simulink model "ramadan_2022"  (R2021a)
settings: Solver=ode15s  StartTime=0.0  StopTime=10  MaxStep=1e-2  MinStep=1e-20  RelTol=1e-3
StartFcn:
  | tic
StopFcn:
  | toc
  | 
  | 
  | %if GimbalLockFlag
  |  % fprintf(2, 'Almost reached Gimbal Lock of IMU. Simulation stopped.\n')
  | %end
  | 
  | %fprintf('Elapsed time: %4.2f sec (%4.2f%% realtime)\n', a, tout(end)/a*100)
values from neighbouring files (symbols this model uses):
  Balance = pMod(26:29)    [AssignSimulinkParams.m]    (also in assign_parameters.m = param(26:29))
  BalanceTrunkLat = pMod(22:25)    [AssignSimulinkParams.m]    (also in assign_parameters.m = param(22:25))
  BasisStim = pMod(1:11)    [AssignSimulinkParams.m]    (also in assign_parameters.m = param(1:11))
  CompliantLeg = pMod(12:14)    [AssignSimulinkParams.m]    (also in assign_parameters.m = param(12:14))
  CompliantLegLat = pMod(15)    [AssignSimulinkParams.m]    (also in assign_parameters.m = param(15))
  lp1 = 0.45    [nms3D_prep.m]
  lp2 = 0.55    [nms3D_prep.m]
  N = size(x,1)    [cmaes_hg.m]
  PreventKneeOverextension = pMod(16:21)    [AssignSimulinkParams.m]    (also in assign_parameters.m = param(16:21))
  propulsion = pMod(35)    [AssignSimulinkParams.m]    (also in assign_parameters.m = param(35))
  s = x(1:N-1,:).^2 + x(2:N,:).^2    [cmaes_hg.m]
  Target02 = pMod(30)    [AssignSimulinkParams.m]    (also in assign_parameters.m = param(30))
  Target13 = pMod(31:33)    [AssignSimulinkParams.m]    (also in assign_parameters.m = param(31:33))
  theta0 = pMod(34)    [AssignSimulinkParams.m]    (also in assign_parameters.m = param(34))
  WramameiSL_1000 = readmatrix('WSL_1000_Norm_Sigmoid_MSE_cont.csv')    [nms3D_prep.m]
  ZramameiSL_1000 = readmatrix('ZSL_1000_Norm_Sigmoid_MSE_cont.csv')    [nms3D_prep.m]
undefined symbols (not defined in the file or in its folder): ICs, mParams, X, Y, Z
libraries: nesl_utility x110, sm_lib x88, simulink x79, eeGeneralControl x28, robotmaniplib x10, dspinverses x10, robotcorelib x5, dspmathops x3, pid_lib x2, vrlib x1
(part 9 of 9)

== system ramadan_2022/Supraspinal Level/Subsystem/Swing Leg/Compute Acceleration Profiles with Minimal Jerk Approach1/Minimal jerk Leg Angle/Minimal Jerk ==
  t : Inport
  a [6x1] : Inport  Port=2
  Add : Sum  Inputs=3
  Constant1 : Constant
  Constant3 : Constant  Value=2
  Demux : Demux  Outputs=6
  Divide3 : Product  Inputs=**
  Divide4 : Product  Inputs=**
  Divide5 : Product  Inputs=**
  Gain : Gain  Gain=60
  Gain1 : Gain  Gain=24
  Gain2 : Gain  Gain=6
  Math Function4 : Math  Operator=pow  SaturateOnIntegerOverflow=on
  Terminator : Terminator
  Terminator1 : Terminator
  Terminator2 : Terminator
  j(t) : Outport
  wires:
  a [6x1]/1 -> Demux/1
  Constant3/1 -> Math Function4/2
  Add/1 -> j(t)/1
  Demux/4 -> Divide3/2
  t/1 -> Divide4/1, Math Function4/1
  Demux/5 -> Divide4/2
  Demux/6 -> Divide5/2
  Demux/1 -> Terminator/1
  Demux/2 -> Terminator1/1
  Divide3/1 -> Gain2/1
  Divide4/1 -> Gain1/1
  Divide5/1 -> Gain/1
  Gain/1 -> Add/3
  Gain1/1 -> Add/2
  Gain2/1 -> Add/1
  Math Function4/1 -> Divide5/1
  Constant1/1 -> Divide3/1
  Demux/3 -> Terminator2/1

== system ramadan_2022/Supraspinal Level/Subsystem/Swing Leg/Compute Acceleration Profiles with Minimal Jerk Approach1/Minimal jerk Leg Angle/Minimal Jerk Parameters [Movellan] ==
  x0 : Inport
  dx0 : Inport  Port=2
  ddx0 : Inport  Port=3
  xT : Inport  Port=4
  dxT : Inport  Port=5
  ddxT : Inport  Port=6
  T : Inport  Port=7
  Demux : Demux  Outputs=3
  Gain : Gain  Gain=0.5
  Gain1 : Gain  Gain=3
  Gain2 : Gain  Gain=6
  Gain3 : Gain  Gain=4
  Gain4 : Gain  Gain=12
  Gain5 : Gain  Gain=5
  Gain6 : Gain  Gain=20
  Matrix Multiply : Product  Multiplication=Matrix(*)
  Minus : Sum  Inputs=+---
  Minus1 : Sum  Inputs=+--
  Minus2 : Sum  Inputs=+-
  Mux : Mux  Inputs=6
  Mux{1..4} (4 alike) : Mux  Inputs=3
  Pseudoinverse : dspinverses/Pseudoinverse  wanterr=off  SimulateUsing=Code generation
      settings: SourceProductBaseCode=DS
  T{2..5} (4 alike) : Product  Inputs=**
  b : Concatenate  NumInputs=3  Mode=Multidimensional array  ConcatenateDimension=2
  multiply : Product  Inputs=**
  multiply1 : Product  Inputs=**
  multiply2 : Product  Inputs=**
  a : Outport
  wires:
  xT/1 -> Minus/1
  Minus1/1 -> Mux4/2
  T5/1 -> Mux3/1
  multiply1/1 -> Minus1/3
  Gain5/1 -> Mux3/2
  Demux/2 -> Mux/5
  dxT/1 -> Minus1/1
  Demux/3 -> Mux/6
  b/1 -> Pseudoinverse/1
  multiply2/1 -> Minus/3
  Minus2/1 -> Mux4/3
  Gain/1 -> multiply/1, Mux/3
  multiply/1 -> Minus/4
  ddxT/1 -> Minus2/1
  Gain4/1 -> Mux2/3
  Gain6/1 -> Mux3/3
  x0/1 -> Minus/2, Mux/1
  Mux1/1 -> b/1
  Matrix Multiply/1 -> Demux/1
  ddx0/1 -> Minus2/2, multiply1/1, Gain/1
  T2/1 -> Gain1/1, Gain4/1, T3/1, multiply/2
  Gain2/1 -> Mux1/3
  Mux4/1 -> Matrix Multiply/2
  T4/1 -> Mux2/1, Gain5/1, T5/1
  Minus/1 -> Mux4/1
  Pseudoinverse/1 -> Matrix Multiply/1
  Mux2/1 -> b/2
  Gain3/1 -> Mux2/2
  Mux3/1 -> b/3
  Gain1/1 -> Mux1/2
  T/1 -> multiply2/2, multiply1/2, Gain2/1, T5/2, T4/2, T3/2, T2/2, T2/1
  Demux/1 -> Mux/4
  Mux/1 -> a/1
  T3/1 -> Gain6/1, Gain3/1, Mux1/1, T4/1
  dx0/1 -> multiply2/1, Minus1/2, Mux/2

== system ramadan_2022/Supraspinal Level/Subsystem/Swing Leg/Compute Acceleration Profiles with Minimal Jerk Approach1/Minimal jerk Leg Length/Enabled Subsystem ==
  In1 : Inport
  Enable : EnablePort
  Out1 : Outport  VectorParamsAs1DForOutWhenUnconnected=off
  wires:
  In1/1 -> Out1/1

== system ramadan_2022/Supraspinal Level/Subsystem/Swing Leg/Compute Acceleration Profiles with Minimal Jerk Approach1/Minimal jerk Leg Length/Minimal Jerk ==
  t : Inport
  a [6x1] : Inport  Port=2
  Add : Sum  Inputs=3
  Constant1 : Constant
  Constant3 : Constant  Value=2
  Demux : Demux  Outputs=6
  Divide3 : Product  Inputs=**
  Divide4 : Product  Inputs=**
  Divide5 : Product  Inputs=**
  Gain : Gain  Gain=60
  Gain1 : Gain  Gain=24
  Gain2 : Gain  Gain=6
  Math Function4 : Math  Operator=pow  SaturateOnIntegerOverflow=on
  Terminator : Terminator
  Terminator1 : Terminator
  Terminator2 : Terminator
  j(t) : Outport
  wires:
  a [6x1]/1 -> Demux/1
  Constant3/1 -> Math Function4/2
  Add/1 -> j(t)/1
  Demux/4 -> Divide3/2
  t/1 -> Divide4/1, Math Function4/1
  Demux/5 -> Divide4/2
  Demux/6 -> Divide5/2
  Demux/1 -> Terminator/1
  Demux/2 -> Terminator1/1
  Divide3/1 -> Gain2/1
  Divide4/1 -> Gain1/1
  Divide5/1 -> Gain/1
  Gain/1 -> Add/3
  Gain1/1 -> Add/2
  Gain2/1 -> Add/1
  Math Function4/1 -> Divide5/1
  Constant1/1 -> Divide3/1
  Demux/3 -> Terminator2/1

== system ramadan_2022/Supraspinal Level/Subsystem/Swing Leg/Compute Acceleration Profiles with Minimal Jerk Approach1/Minimal jerk Leg Length/Minimal Jerk Parameters [Movellan] ==
  x0 : Inport
  dx0 : Inport  Port=2
  ddx0 : Inport  Port=3
  xT : Inport  Port=4
  dxT : Inport  Port=5
  ddxT : Inport  Port=6
  T : Inport  Port=7
  Demux : Demux  Outputs=3
  Gain : Gain  Gain=0.5
  Gain1 : Gain  Gain=3
  Gain2 : Gain  Gain=6
  Gain3 : Gain  Gain=4
  Gain4 : Gain  Gain=12
  Gain5 : Gain  Gain=5
  Gain6 : Gain  Gain=20
  Matrix Multiply : Product  Multiplication=Matrix(*)
  Minus : Sum  Inputs=+---
  Minus1 : Sum  Inputs=+--
  Minus2 : Sum  Inputs=+-
  Mux : Mux  Inputs=6
  Mux{1..4} (4 alike) : Mux  Inputs=3
  Pseudoinverse : dspinverses/Pseudoinverse  wanterr=off  SimulateUsing=Code generation
      settings: SourceProductBaseCode=DS
  T{2..5} (4 alike) : Product  Inputs=**
  b : Concatenate  NumInputs=3  Mode=Multidimensional array  ConcatenateDimension=2
  multiply : Product  Inputs=**
  multiply1 : Product  Inputs=**
  multiply2 : Product  Inputs=**
  a : Outport
  wires:
  xT/1 -> Minus/1
  Minus1/1 -> Mux4/2
  T5/1 -> Mux3/1
  multiply1/1 -> Minus1/3
  Gain5/1 -> Mux3/2
  Demux/2 -> Mux/5
  dxT/1 -> Minus1/1
  Demux/3 -> Mux/6
  b/1 -> Pseudoinverse/1
  multiply2/1 -> Minus/3
  Minus2/1 -> Mux4/3
  Gain/1 -> multiply/1, Mux/3
  multiply/1 -> Minus/4
  ddxT/1 -> Minus2/1
  Gain4/1 -> Mux2/3
  Gain6/1 -> Mux3/3
  x0/1 -> Minus/2, Mux/1
  Mux1/1 -> b/1
  Matrix Multiply/1 -> Demux/1
  ddx0/1 -> Minus2/2, multiply1/1, Gain/1
  T2/1 -> Gain1/1, Gain4/1, T3/1, multiply/2
  Gain2/1 -> Mux1/3
  Mux4/1 -> Matrix Multiply/2
  T4/1 -> Mux2/1, Gain5/1, T5/1
  Minus/1 -> Mux4/1
  Pseudoinverse/1 -> Matrix Multiply/1
  Mux2/1 -> b/2
  Gain3/1 -> Mux2/2
  Mux3/1 -> b/3
  Gain1/1 -> Mux1/2
  T/1 -> multiply2/2, multiply1/2, Gain2/1, T5/2, T4/2, T3/2, T2/2, T2/1
  Demux/1 -> Mux/4
  Mux/1 -> a/1
  T3/1 -> Gain6/1, Gain3/1, Mux1/1, T4/1
  dx0/1 -> multiply2/1, Minus1/2, Mux/2

== system ramadan_2022/Supraspinal Level/Subsystem/Swing Leg/Inverse Dynamics: Left Leg/Inverse Dynamics/Inverse Dynamics ==
  note: Inverse Dynamics: This block computes the 14 torques (joints(8), body rotation(3) and body translation(3)) needed to generate the desired joint accelerations compensating inertial, velocity depended and gravitational torques at the same time.
  Config : Inport
  JointVel : Inport  Port=2
  Des. JointAccel : Inport  Port=3
  Real JointAccel : Inport  Port=4
  Add : Sum  Inputs=+++
  Gravity Torque : robotmaniplib/Gravity Torque  RigidBodyTree=model_swing_left  SimulateUsing=Code generation
  Joint Space Mass Matrix : robotmaniplib/Joint Space Mass Matrix  RigidBodyTree=model_swing_left  SimulateUsing=Code generation
  Matrix Multiply : Product  Multiplication=Matrix(*)
  Matrix Multiply1 : Product  Multiplication=Matrix(*)
  Select Body Joint Torques : Selector  InputPortWidth=10  IndexOptions=Index vector (dialog)  Indices=[7:10]  OutputSizes=1
  Select Wrench2 : Selector  InputPortWidth=10  IndexOptions=Index vector (dialog)  Indices=[1 2 3 4 5 6]  OutputSizes=1
  Velocity Product Torque : robotmaniplib/Velocity Product Torque  RigidBodyTree=model_swing_left  SimulateUsing=Code generation
      settings: SourceProductBaseCode=RO
  Desired Torques : Outport  VectorParamsAs1DForOutWhenUnconnected=off
  Interaction Wrench Left : Outport  Port=2  VectorParamsAs1DForOutWhenUnconnected=off
  wires:
  Add/1 -> Select Body Joint Torques/1
  Select Body Joint Torques/1 -> Desired Torques/1
  Config/1 -> Joint Space Mass Matrix/1, Gravity Torque/1, Velocity Product Torque/1
  JointVel/1 -> Velocity Product Torque/2
  Des. JointAccel/1 -> Matrix Multiply/2
  Gravity Torque/1 -> Add/2
  Select Wrench2/1 -> Interaction Wrench Left/1
  Matrix Multiply1/1 -> Select Wrench2/1
  Joint Space Mass Matrix/1 -> Matrix Multiply1/1, Matrix Multiply/1
  Matrix Multiply/1 -> Add/1
  Velocity Product Torque/1 -> Add/3
  Real JointAccel/1 -> Matrix Multiply1/2

== system ramadan_2022/Supraspinal Level/Subsystem/Swing Leg/Inverse Dynamics: Right Leg/Inverse Dynamics1/Inverse Dynamics ==
  note: Inverse Dynamics: This block computes the 14 torques (joints(8), body rotation(3) and body translation(3)) needed to generate the desired joint accelerations compensating inertial, velocity depended and gravitational torques at the same time.
  Config : Inport
  JointVel : Inport  Port=2
  Des. JointAccel : Inport  Port=3
  Real JointAccel : Inport  Port=4
  Add : Sum  Inputs=+++
  Gravity Torque : robotmaniplib/Gravity Torque  RigidBodyTree=model_swing_right  SimulateUsing=Code generation
  Joint Space Mass Matrix : robotmaniplib/Joint Space Mass Matrix  RigidBodyTree=model_swing_right  SimulateUsing=Code generation
  Matrix Multiply : Product  Multiplication=Matrix(*)
  Matrix Multiply1 : Product  Multiplication=Matrix(*)
  Select Body Joint Torques : Selector  InputPortWidth=10  IndexOptions=Index vector (dialog)  Indices=[7:10]  OutputSizes=1
  Select Wrench2 : Selector  InputPortWidth=10  IndexOptions=Index vector (dialog)  Indices=[1 2 3 4 5 6]  OutputSizes=1
  Velocity Product Torque : robotmaniplib/Velocity Product Torque  RigidBodyTree=model_swing_right  SimulateUsing=Code generation
      settings: SourceProductBaseCode=RO
  Desired Torques : Outport  VectorParamsAs1DForOutWhenUnconnected=off
  Interaction Wrench Left : Outport  Port=2  VectorParamsAs1DForOutWhenUnconnected=off
  wires:
  Add/1 -> Select Body Joint Torques/1
  Select Body Joint Torques/1 -> Desired Torques/1
  JointVel/1 -> Velocity Product Torque/2
  Des. JointAccel/1 -> Matrix Multiply/2
  Gravity Torque/1 -> Add/2
  Select Wrench2/1 -> Interaction Wrench Left/1
  Matrix Multiply1/1 -> Select Wrench2/1
  Joint Space Mass Matrix/1 -> Matrix Multiply1/1, Matrix Multiply/1
  Matrix Multiply/1 -> Add/1
  Velocity Product Torque/1 -> Add/3
  Config/1 -> Joint Space Mass Matrix/1, Gravity Torque/1, Velocity Product Torque/1
  Real JointAccel/1 -> Matrix Multiply1/2

== stateflow chart ramadan_2022/Supraspinal Level/Finite State Machine/Chart ==
  settings: executeAtInitialization=1
  state State0
    entry:
    state0=1;
    state1=0;
    state2=0;
    state3=0;
    state4=0;
    state5=0;
  state State1
    entry:
    state0=0;
    state1=1;
    state2=0;
    state3=0;
    state4=0;
    state5=0;
  state State5
    entry:
    state0=0;
    state1=0;
    state2=0;
    state3=0;
    state4=0;
    state5=1;
  state State4
    entry:
    state0=0;
    state1=0;
    state2=0;
    state3=0;
    state4=1;
    state5=0;
  state State3
    entry:
    state0=0;
    state1=0;
    state2=0;
    state3=1;
    state4=0;
    state5=0;
  state State2
    entry:
    state0=0;
    state1=0;
    state2=1;
    state3=0;
    state4=0;
    state5=0;
  (default) -> State0
  State1 -> State4 [order 2] : after(lp2*dt,sec)
  State0 -> State1 : after(lp1*dt,sec)
  State3 -> State0 [order 1] : [contact_left]
  State1 -> State2 [order 1] : [contact_right]
  State3 -> State5 [order 2] : after(lp2*dt,sec)
  State4 -> State2 : [contact_right]
  State2 -> State3 : after(lp1*dt,sec)
  data: lp2 input; lp1 input; state0 output; state1 output; state2 output; state3 output; dt input; contact_left input; contact_right input; state4 output; state5 output
